simulink library "Power_Shaft2_Electric_L1_R1"  (R2022a)
settings: Solver=VariableStepAuto  StartTime=0.0  StopTime=10.0  RelTol=1e-3
values from neighbouring files (symbols this model uses):
  VDatabase = evalin('base','VDatabase')    [sm_car_controlparam_Electric_A1_A2_default.m]
undefined symbols (not defined in the file or in its folder): ShaftL1, ShaftR1
libraries: Power_Components x3, fl_lib x2, sm_lib x1, Cooling_Motor2_L1R1 x1
Description:
  | Component of Simscape Vehicle Templates Library
  | 
  | Copyright 2018-2024 The MathWorks, Inc.
settings Model: Creator=smiller  LastModifiedBy=smiller
settings SolverCC: AlgebraicLoopSolver=TrustRegion
settings DataIOCC: ReturnWorkspaceOutputs=off
settings DebuggingCC: UnconnectedInputMsg=warning  UnconnectedOutputMsg=warning  UnconnectedLineMsg=warning  SFMachineParentedDataDiag=warning  ArithmeticOperatorsInVariantConditions=warning
settings SFSimCC: CustomCodeUndefinedFunction=UseInterfaceOnly

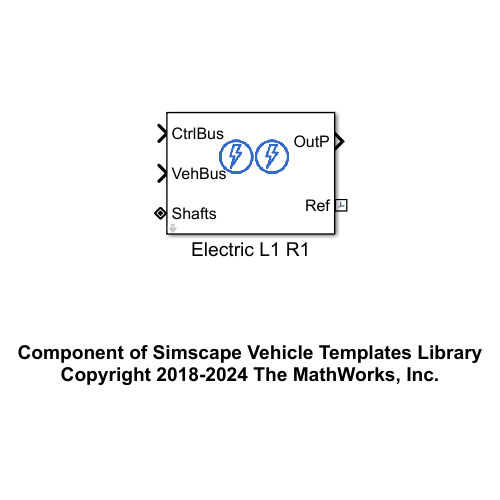
[thumbnail: Simulink's stored preview of the top-level diagram]
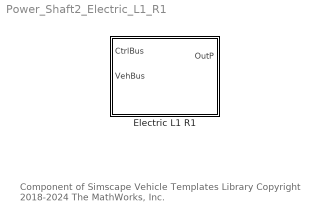
== system Power_Shaft2_Electric_L1_R1 ==
  note: Component of Simscape Vehicle Templates Library
      | Copyright 2018-2024 The MathWorks, Inc.
  Electric L1 R1 : Subsystem  mask(Electric Propulsion with Two Motors){Power=VDatabase.Power.Electric2Motor_L1_R1_default}
      mask prompts: Power "Power 4 Motor (structure)"
      mask help: Two electric motors with optional cooling system. Physical connections for the two motor shafts are in bus Shafts and connect to the front left and front right wheels.
      mask Display: image('sm_car_vehicle_power_e2motor_L1R1_IMAGE.png');

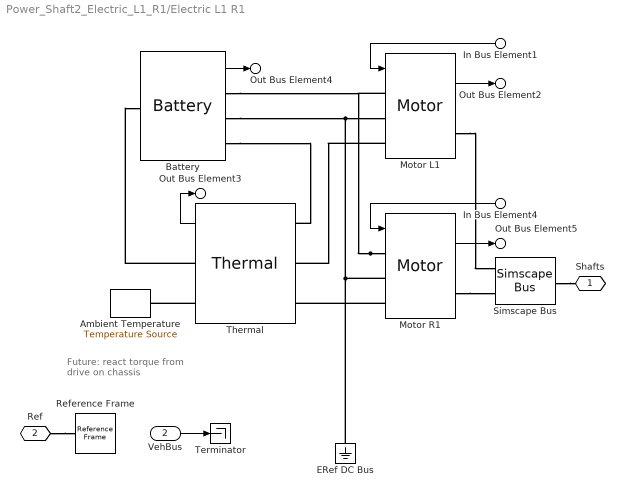
== system Power_Shaft2_Electric_L1_R1/Electric L1 R1 ==
  note: Future:
      | react torque
      | from drive
      | on chassis
  In Bus Element1 : Inport  PortName=CtrlBus  Element=MMotorL1Demand
  In Bus Element4 : Inport  PortName=CtrlBus  Element=MMotorR1Demand
  VehBus : Inport  Port=2
  Ambient Temperature : fl_lib/Thermal/Thermal Sources/Temperature Source  temperature=Power.TAmbient.Value K
      settings: SourceProductBaseCode=PW,SS,VE
  Battery : Power_Components/Battery  SystemSampleTime=-1  VariantActivationTime=update diagram  Latency=0  AutoFrameSizeCalculation=off
  ERef DC Bus : fl_lib/Electrical/Electrical Elements/Electrical Reference
      settings: SourceProductBaseCode=PW,SS,VE
  Motor L1 : Power_Components/Motor  Motor=Power.MotorL1
  Motor R1 : Power_Components/Motor  Motor=Power.MotorL1
  Reference Frame : sm_lib/Frames and Transforms/Reference Frame
  Simscape Bus : SimscapeBus  HierarchyStrings=ShaftL1;ShaftR1
  Terminator : Terminator
  Thermal : Cooling_Motor2_L1R1/Thermal  VariantControl=Variant1  LabelModeActiveChoice=Liquid_Loop1  VariantLabel=Power.Cooling.class.Value
      settings: AttributesFormatString=%<ActiveVariant>
  Shafts : PMIOPort  Side=Left
  Ref : PMIOPort  Port=2  Side=Right
  Out Bus Element2 : Outport  VectorParamsAs1DForOutWhenUnconnected=off  PortName=OutP  Element=MotorL1
  Out Bus Element3 : Outport  VectorParamsAs1DForOutWhenUnconnected=off  PortName=OutP  Element=Thermal
  Out Bus Element4 : Outport  VectorParamsAs1DForOutWhenUnconnected=off  PortName=OutP  Element=Battery
  Out Bus Element5 : Outport  VectorParamsAs1DForOutWhenUnconnected=off  PortName=OutP  Element=MotorR1
  wires:
  In Bus Element1/1 -> Motor L1/1
  Motor L1/1 -> Out Bus Element2/1
  Thermal/1 -> Out Bus Element3/1
  VehBus/1 -> Terminator/1
  Battery/1 -> Out Bus Element4/1
  Motor R1/1 -> Out Bus Element5/1
  In Bus Element4/1 -> Motor R1/1
  connections:
  ERef DC Bus/LConn1 -- Battery/RConn2 -- Motor L1/LConn2 -- Motor R1/LConn2
  Motor R1/LConn1 -- Battery/RConn1 -- Motor L1/LConn1
  Motor L1/RConn1 -- Simscape Bus/LConn1
  Simscape Bus/RConn1 -- Shafts/RConn1
  Ref/RConn1 -- Reference Frame/RConn1
  Motor L1/LConn3 -- Thermal/LConn2
  Thermal/RConn2 -- Ambient Temperature/LConn1
  Battery/RConn3 -- Thermal/LConn1
  Thermal/RConn1 -- Battery/LConn1
  Motor R1/RConn1 -- Simscape Bus/LConn2
  Motor R1/LConn3 -- Thermal/LConn3
